simulink model "Simulator"  (R2024a)
settings: Solver=VariableStepAuto  StartTime=0.0  StopTime=inf  RelTol=1e-5
values from neighbouring files (symbols this model uses):
  I = [3000 0 0 ... (first row only)    [Constants_gui.m]    (also in constants.m; mbi.m = [15, .25, .20; set_up_HW7.m = I-Id; setupConstantRateSDA.m)
  invI = inv(I)    [Constants_gui.m]    (also in constants.m; mbi.m; set_up_HW7.m; setupConstantRateSDA.m)
  q_init = q_init/norm(q_init)    [Constants_gui.m]    (also in constants.m = [-0.5 -0.5 -0.5 0.5]; mbi.m = [0 0 0 1]'; set_up_HW7.m = [0 0 0 1]'; setupConstantRateSDA.m)
  wbn_init = pi/30*[0 0 0]'    [Constants_gui.m]    (also in constants.m = pi/180 * [0.1; 0.2; 0.15]; mbi.m = [0 0 0]'; set_up_HW7.m = pi/30*[0 0 .01]'; setupConstantRateSDA.m)
  wn = 0.01    [Constants_gui.m]    (also in constants.m = 0.05; setupConstantRateSDA.m = 0.05)
  zet = .7071    (= 0.7071)    [Constants_gui.m]    (also in constants.m; setupConstantRateSDA.m)
undefined symbols (not defined in the file or in its folder): w_init
libraries: sharedtransform x6, aerolibutil x5, sharedutil x2, simulink x2, dspinverses x1
(part 3 of 4)

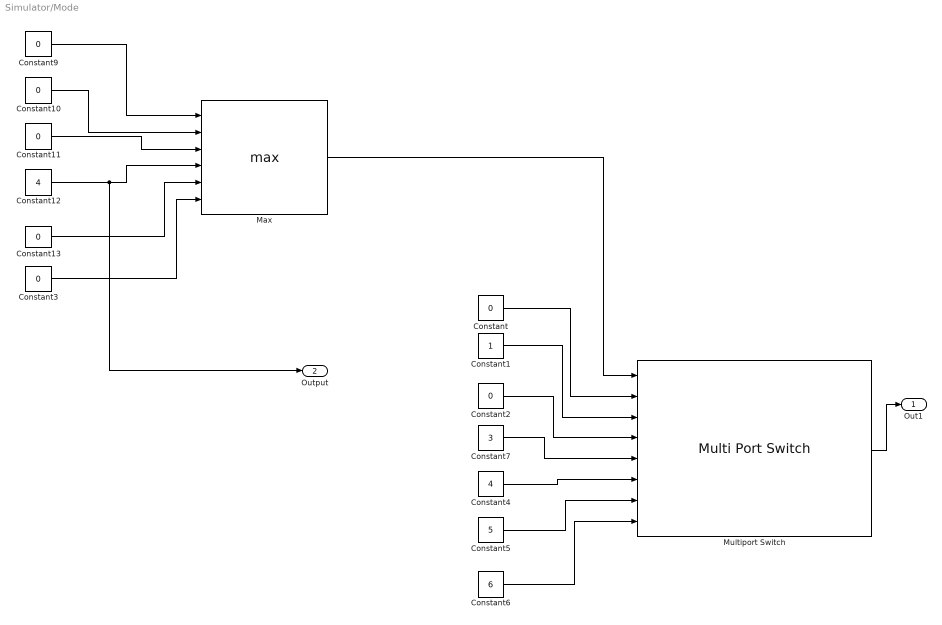
== system Simulator/Mode ==
  Constant{,2..3,9..11,13} (7 alike) : Constant  Value=0
  Constant1 : Constant
  Constant12 : Constant  Value=4
  Constant4 : Constant  Value=4
  Constant5 : Constant  Value=5
  Constant6 : Constant  Value=6
  Constant7 : Constant  Value=3
  Max : MinMax  Function=max  Inputs=6
  Multiport Switch : MultiPortSwitch  DataPortOrder=Specify indices  Inputs=6  DataPortIndices={0,1,2,3,4,5,6}  SaturateOnIntegerOverflow=off  InputSameDT=off
  Out1 : Outport
  Output : Outport  Port=2
  wires:
  Multiport Switch/1 -> Out1/1
  Constant6/1 -> Multiport Switch/8
  Constant5/1 -> Multiport Switch/7
  Constant4/1 -> Multiport Switch/6
  Constant7/1 -> Multiport Switch/5
  Constant2/1 -> Multiport Switch/4
  Constant1/1 -> Multiport Switch/3
  Constant/1 -> Multiport Switch/2
  Constant9/1 -> Max/1
  Constant10/1 -> Max/2
  Constant11/1 -> Max/3
  Constant12/1 -> Output/1, Max/4
  Constant13/1 -> Max/5
  Constant3/1 -> Max/6
  Max/1 -> Multiport Switch/1

== system Simulator/Mode 0  ==
  In1 : Inport
  In2 : Inport  Port=2
  Q : Inport  Port=3
  Rate : Inport  Port=4
  Commanded Quaternion : Subsystem
  Constant : Constant
  Switch : Switch  Criteria=u2 > Threshold  SaturateOnIntegerOverflow=off  InputSameDT=off
  Rate2 : Outport
  Quaternion : Outport  Port=2
  wires:
  Rate/1 -> Rate2/1
  Switch/1 -> Quaternion/1
  Constant/1 -> Switch/2
  Q/1 -> Switch/3
  Commanded Quaternion/1(QUaternion) -> Switch/1

== system Simulator/Mode 1: Full Test ==
  In1 : Inport
  Out1 : Outport
  Out2 : Outport  Port=2
  wires:
  In1/1 -> Out2/1, Out1/1

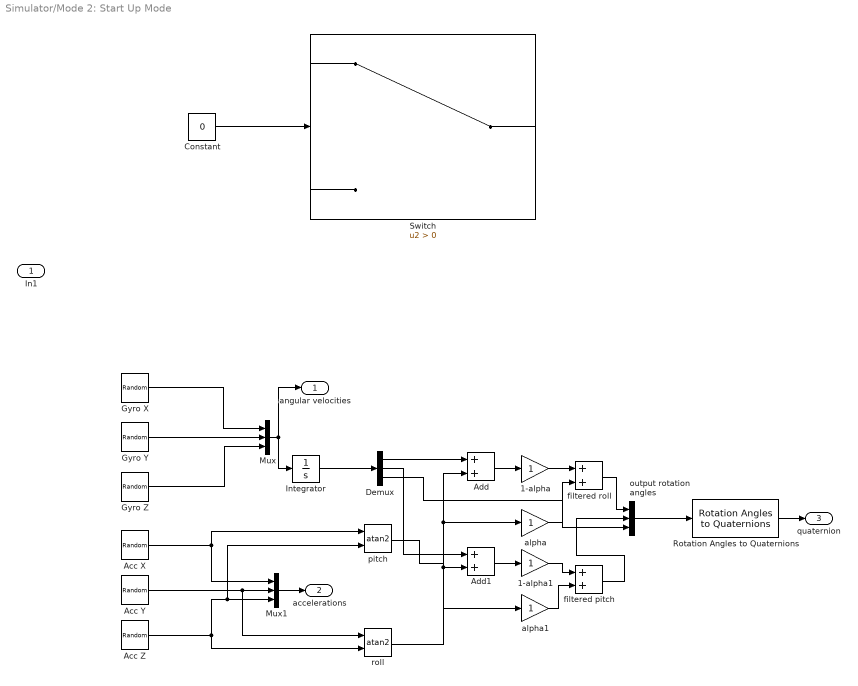
== system Simulator/Mode 2: Start Up Mode ==
  In1 : Inport
  1-alpha : Gain
  1-alpha1 : Gain
  Acc X : UniformRandomNumber  Minimum=w_init  Maximum=100  SampleTime=0.1
  Acc Y : UniformRandomNumber  Minimum=w_init  Maximum=100  SampleTime=0.1
  Acc Z : UniformRandomNumber  Minimum=w_init  Maximum=100  SampleTime=0.1
  Add : Sum
  Add1 : Sum
  Constant : Constant  Value=0
  Demux : Demux  Outputs=3
  Gyro X : UniformRandomNumber  Minimum=w_init  Maximum=100  SampleTime=0.1
  Gyro Y : UniformRandomNumber  Minimum=w_init  Maximum=100  SampleTime=0.1
  Gyro Z : UniformRandomNumber  Minimum=w_init  Maximum=100  SampleTime=0.1
  Integrator : Integrator
  Mux : Mux  Inputs=3
  Mux1 : Mux  Inputs=3
  Rotation Angles to Quaternions : sharedtransform/Rotation Angles to Quaternions  rotationOrder=XYZ  aMode=aMode
  Switch : Switch  Criteria=u2 > Threshold  SaturateOnIntegerOverflow=off  InputSameDT=off
  alpha : Gain
  alpha1 : Gain
  filtered pitch : Sum
  filtered roll : Sum
  output rotation angles : Mux  Inputs=3
  pitch : Trigonometry  Operator=atan2
  roll : Trigonometry  Operator=atan2
  angular velocities : Outport
  accelerations : Outport  Port=2
  quaternion : Outport  Port=3
  wires:
  Gyro X/1 -> Mux/1
  Gyro Y/1 -> Mux/2
  Gyro Z/1 -> Mux/3
  Mux/1 -> Integrator/1, angular velocities/1
  Mux1/1 -> accelerations/1
  Acc X/1 -> pitch/1, Mux1/1
  Acc Y/1 -> Mux1/2, roll/1
  Acc Z/1 -> roll/2, Mux1/3, pitch/2
  Integrator/1 -> Demux/1
  Demux/3 -> output rotation angles/3
  Demux/1 -> Add/1
  roll/1 -> alpha/1, Add/2
  Add/1 -> 1-alpha/1
  1-alpha/1 -> filtered roll/1
  alpha/1 -> filtered roll/2
  Demux/2 -> Add1/1
  pitch/1 -> Add1/2, alpha1/1
  Add1/1 -> 1-alpha1/1
  1-alpha1/1 -> filtered pitch/1
  alpha1/1 -> filtered pitch/2
  filtered roll/1 -> output rotation angles/1
  filtered pitch/1 -> output rotation angles/2
  output rotation angles/1 -> Rotation Angles to Quaternions/1
  Rotation Angles to Quaternions/1 -> quaternion/1
  Constant/1 -> Switch/2

== system Simulator/Mode 3: Constant Rate ==
  rotation rate mode : Inport
  commanded Velocity : Inport  Port=2
  "Free Rigid Body " : Subsystem
  Kd1 : Gain  Gain=2 * zet * wn * I  Multiplication=Matrix(K*u)  SaturateOnIntegerOverflow=on  OutDataTypeStr=Inherit: Same as input  ParamDataTypeStr=Inherit: Same as input
  Sum1 : Sum  Inputs=|+-
  rotation rate : Outport
  "quaat " : Outport  Port=2
  wires:
  Kd1/1 -> "Free Rigid Body "/1(In2)
  Sum1/1 -> Kd1/1
  "Free Rigid Body "/2(w) -> rotation rate/1, Sum1/2
  "Free Rigid Body "/1(q) -> "quaat "/1
  commanded Velocity/1 -> Sum1/1

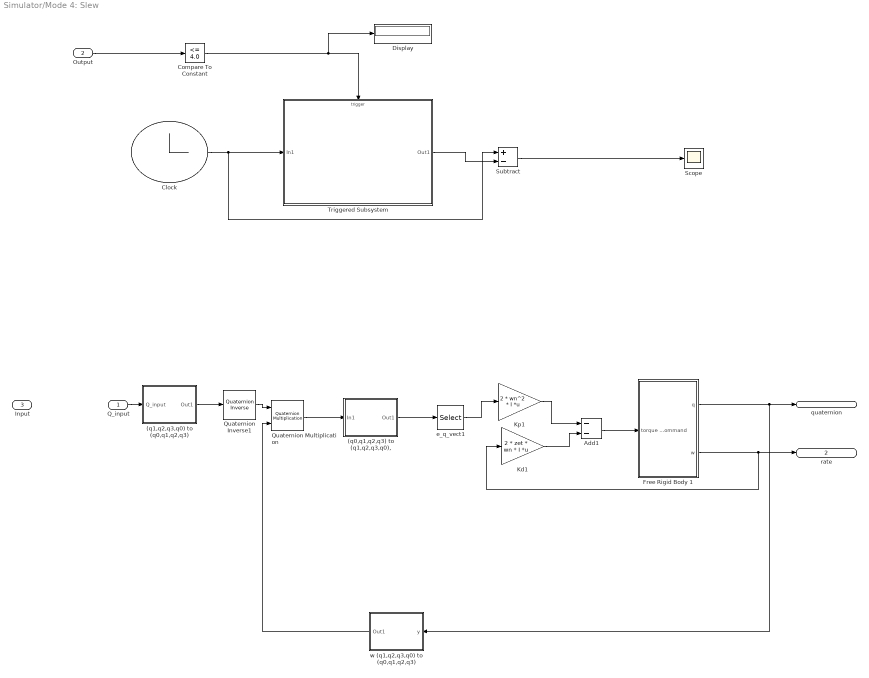
== system Simulator/Mode 4: Slew ==
  Q_input : Inport
  Output : Inport  Port=2
  " Input" : Inport  Port=3
  (q0,q1,q2,q3) to (q1,q2,q3,q0), : Subsystem
  "(q1,q2,q3,q0) to (q0,q1,q2,q3) " : Subsystem
  Add1 : Sum  Inputs=--
  Clock : Clock
  Compare To Constant : simulink/Logic and Bit Operations/Compare To Constant  relop=<=  const=4.0  OutDataTypeStr=boolean
  Display : Display
  Free Rigid Body 1 : Subsystem
  Kd1 : Gain  Gain=2 * zet * wn * I  Multiplication=Matrix(K*u)  SaturateOnIntegerOverflow=on  OutDataTypeStr=Inherit: Same as input  ParamDataTypeStr=Inherit: Same as input
  Kp1 : Gain  Gain=2 * wn^2 * I  Multiplication=Matrix(K*u)  SaturateOnIntegerOverflow=on  OutDataTypeStr=Inherit: Same as input  ParamDataTypeStr=Inherit: Same as input
  Quaternion Inverse1 : aerolibutil/Quaternion Inverse
  Quaternion Multiplication : aerolibutil/Quaternion Multiplication
  Scope : Scope
  Subtract : Sum  Inputs=+-
  Triggered Subsystem : Subsystem  TreatAsAtomicUnit=on
  e_q_vect1 : Selector  InputPortWidth=4  IndexOptions=Index vector (dialog)  Indices=[1 2 3]  OutputSizes=1
  "w (q1,q2,q3,q0) to (q0,q1,q2,q3) " : Subsystem
      settings: PortSchema="{\"entries\":[{\"content\":{\"sides\":[{\"content\":{\"connectorIds\":[\"Out1\"]},\"type\":\"ConnectorPlacement.EquallySpacedRectSide\",\"uuid\":\"97b477ad-5663-4010-b344-d27b8ec095be\"},{\"content\":{\"connectorIds\":[\"In1\"],\"side\":\"RIGHT\"},\"type\":\"ConnectorPlacement.EquallySpacedRectSide\",\"uuid\":\"41fe4029-0263-4427-bdfc-3c26258b8a65\"},{\"content\":{\"side\":\"TOP\"},\"type\":\"ConnectorPlacement.EquallySpacedRectSide\",\"uuid\":\"9fb3a03d-539a-4245-bd7d-8174d3d0797f\"}]},\"type\":\"ConnectorPlacement.EquallySpacedConnector\",\"uuid\":\"44222554-f3ae-4bc6-b92c-7571a5ce84f7\"}],\"packageUris\":[\"http://schema.mathworks.com/mf0/Connector/R2020b\"],\"version\":\"1.0\"}"
  quaternion : Outport
  rate : Outport  Port=2
  wires:
  Free Rigid Body 1/2(w) -> rate/1, Kd1/1
  Quaternion Inverse1/1 -> Quaternion Multiplication/1
  (q0,q1,q2,q3) to (q1,q2,q3,q0),/1(Out1) -> e_q_vect1/1
  Quaternion Multiplication/1 -> (q0,q1,q2,q3) to (q1,q2,q3,q0),/1(In1)
  Add1/1 -> Free Rigid Body 1/1(torque command)
  "w (q1,q2,q3,q0) to (q0,q1,q2,q3) "/1(Out1) -> Quaternion Multiplication/2
  "(q1,q2,q3,q0) to (q0,q1,q2,q3) "/1(Out1) -> Quaternion Inverse1/1
  Kd1/1 -> Add1/2
  Free Rigid Body 1/1(q) -> quaternion/1, "w (q1,q2,q3,q0) to (q0,q1,q2,q3) "/1(y)
  e_q_vect1/1 -> Kp1/1
  Kp1/1 -> Add1/1
  Q_input/1 -> "(q1,q2,q3,q0) to (q0,q1,q2,q3) "/1(Q_input)
  Clock/1 -> Subtract/1, Triggered Subsystem/1(In1)
  Output/1 -> Compare To Constant/1
  Compare To Constant/1 -> Display/1, Triggered Subsystem/Trigger
  Triggered Subsystem/1(Out1) -> Subtract/2
  Subtract/1 -> Scope/1

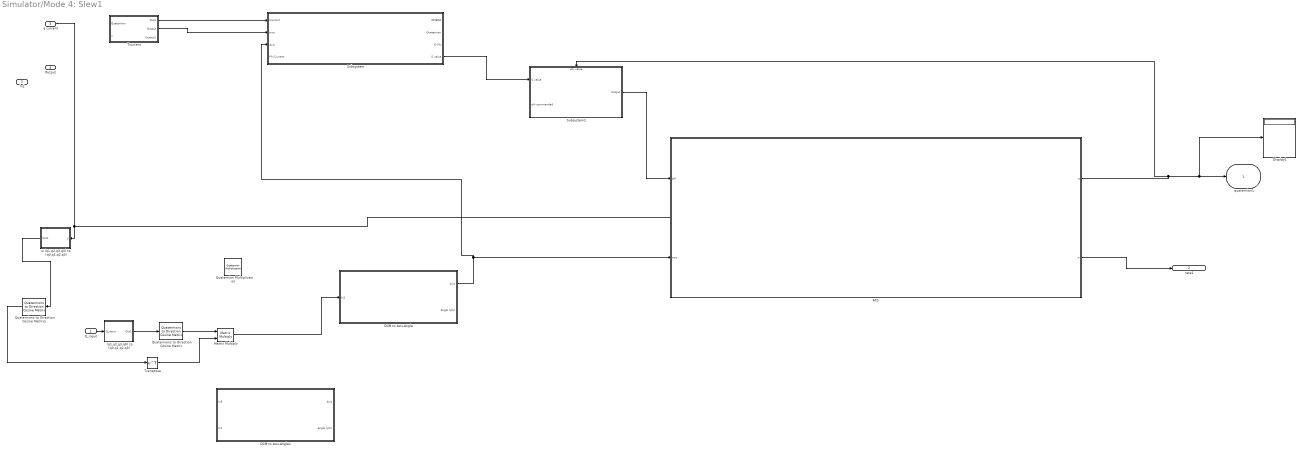
== system Simulator/Mode 4: Slew1 ==
  Q_input : Inport
  In2 : Inport  Port=2
  q current : Inport  Port=3
  Output : Inport  Port=4
  "(q1,q2,q3,q0) to (q0,q1,q2,q3) " : Subsystem
  ACS : Subsystem
  DCM to Axis-Angle : Subsystem
  DCM to Axis-Angle1 : Subsystem
  Display1 : Display
  Matrix Multiply : Product  Multiplication=Matrix(*)
  Quaternion Multiplication : aerolibutil/Quaternion Multiplication
  Quaternions to Direction Cosine Matrix : sharedtransform/Quaternions to  Direction Cosine Matrix  aMode=aMode
      settings: LibrarySourceBlock=|
      | aerolibtransform2/Quaternions to
      | Direction Cosine Matrix
  Quaternions to Direction Cosine Matrix1 : sharedtransform/Quaternions to  Direction Cosine Matrix  aMode=aMode
      settings: LibrarySourceBlock=|
      | aerolibtransform2/Quaternions to
      | Direction Cosine Matrix
  Subsystem : Subsystem
  Subsystem2 : Subsystem
      settings: PortSchema="{\"entries\":[{\"content\":{\"sides\":[{\"content\":{\"connectorIds\":[\"In1\",\"In2\"]},\"type\":\"ConnectorPlacement.EquallySpacedRectSide\",\"uuid\":\"d1e910e7-02fe-476a-80f5-06936a5c67bc\"},{\"content\":{\"connectorIds\":[\"Out1\"],\"side\":\"RIGHT\"},\"type\":\"ConnectorPlacement.EquallySpacedRectSide\",\"uuid\":\"f2ee99f2-c038-4b18-8075-388ccc728d71\"},{\"content\":{\"connectorIds\":[\"In3\"],\"side\":\"TOP\"},\"type\":\"ConnectorPlacement.EquallySpacedRectSide\",\"uuid\":\"7923cf94-d68b-4fff-9236-03f2ad3fb038\"}]},\"type\":\"ConnectorPlacement.EquallySpacedConnector\",\"uuid\":\"859f0eee-a4bc-4454-90a5-75b168cd4378\"}],\"packageUris\":[\"http://schema.mathworks.com/mf0/Connector/R2020b\"],\"version\":\"1.0\"}"
  Tcurrent : Subsystem
  Transpose : Math  Operator=transpose
  "w (q1,q2,q3,q0) to (q0,q1,q2,q3) " : Subsystem
      settings: PortSchema="{\"entries\":[{\"content\":{\"sides\":[{\"content\":{\"connectorIds\":[\"Out1\"]},\"type\":\"ConnectorPlacement.EquallySpacedRectSide\",\"uuid\":\"97b477ad-5663-4010-b344-d27b8ec095be\"},{\"content\":{\"connectorIds\":[\"In1\"],\"side\":\"RIGHT\"},\"type\":\"ConnectorPlacement.EquallySpacedRectSide\",\"uuid\":\"41fe4029-0263-4427-bdfc-3c26258b8a65\"},{\"content\":{\"side\":\"TOP\"},\"type\":\"ConnectorPlacement.EquallySpacedRectSide\",\"uuid\":\"9fb3a03d-539a-4245-bd7d-8174d3d0797f\"}]},\"type\":\"ConnectorPlacement.EquallySpacedConnector\",\"uuid\":\"44222554-f3ae-4bc6-b92c-7571a5ce84f7\"}],\"packageUris\":[\"http://schema.mathworks.com/mf0/Connector/R2020b\"],\"version\":\"1.0\"}"
  quaternion1 : Outport
  rate1 : Outport  Port=2
  wires:
  Q_input/1 -> "(q1,q2,q3,q0) to (q0,q1,q2,q3) "/1(Q_input)
  Transpose/1 -> Matrix Multiply/2
  "w (q1,q2,q3,q0) to (q0,q1,q2,q3) "/1(Out1) -> Quaternions to Direction Cosine Matrix1/1
  Tcurrent/1(Out1) -> Subsystem/1(tcurrent)
  Tcurrent/2(Output) -> Subsystem/2(tnot)
  Quaternions to Direction Cosine Matrix/1 -> Matrix Multiply/1
  Matrix Multiply/1 -> DCM to Axis-Angle/1(In1)
  DCM to Axis-Angle/1(Axis) -> Subsystem/3(Axis), ACS/2(axis)
  Quaternions to Direction Cosine Matrix1/1 -> Transpose/1
  ACS/1(q) -> Subsystem2/3(phi value), Display1/1, quaternion1/1
  ACS/2(w) -> rate1/1
  q current/1 -> "w (q1,q2,q3,q0) to (q0,q1,q2,q3) "/1(y)
  Subsystem/4(S value) -> Subsystem2/1(S value)
  "(q1,q2,q3,q0) to (q0,q1,q2,q3) "/1(Out1) -> Quaternions to Direction Cosine Matrix/1
  Subsystem2/1(Output) -> ACS/1(phi)
  ? -> DCM to Axis-Angle1/1(In3)
  ? -> DCM to Axis-Angle1/2(In1)

== system Simulator/Mode 5: Attitude Control ==
  In2 : Inport
  Q_input : Inport  Port=2
  Add : Sum  Inputs=+-
  "Free Rigid Body " : Subsystem
  Kd : Gain  Gain=2 * zet * wn * I  Multiplication=Matrix(K*u)  SaturateOnIntegerOverflow=on  OutDataTypeStr=Inherit: Same as input  ParamDataTypeStr=Inherit: Same as input
  Kp : Gain  Gain=2 * wn^2 * I  Multiplication=Matrix(K*u)  SaturateOnIntegerOverflow=on  OutDataTypeStr=Inherit: Same as input  ParamDataTypeStr=Inherit: Same as input
  Sum : Sum  Inputs=|+-
  e_q_vect : Selector  InputPortWidth=4  IndexOptions=Index vector (dialog)  Indices=[1 2 3]  OutputSizes=1
  quaternion : Outport
  rate : Outport  Port=2
  wires:
  Kp/1 -> Add/1
  Sum/1 -> e_q_vect/1
  "Free Rigid Body "/1(q) -> quaternion/1, Sum/2
  e_q_vect/1 -> Kp/1
  Kd/1 -> Add/2
  "Free Rigid Body "/2(w) -> rate/1, Kd/1
  Add/1 -> "Free Rigid Body "/1(torque command)
  Q_input/1 -> Sum/1

== system Simulator/Mode 6: Momentum Dump ==
  In1 : Inport
  In2 : Inport  Port=2
  Cross : Subsystem
  F_thrusters : Constant
  Gain : Gain  Gain=-1
  I_sc : Constant  Value=I
  Matrix Divide : Product  Inputs=*/  Multiplication=Matrix(*)
  current angular momentum : Product  Multiplication=Matrix(*)
  r_thrusters : Constant
  commanded thrust time : Outport
  wires:
  I_sc/1 -> current angular momentum/1
  Gain/1 -> Matrix Divide/1
  Cross/1(AxB) -> Matrix Divide/2
  Matrix Divide/1 -> commanded thrust time/1
  current angular momentum/1 -> Gain/1
  In2/1 -> current angular momentum/2
  r_thrusters/1 -> Cross/1(A)
  F_thrusters/1 -> Cross/2(B)

== system Simulator/Subsystem ==
  q : Inport
  " 1" : Demux  Outputs=3
      settings: DisplayOption=none
  " 2" : Demux  Outputs=3
      settings: DisplayOption=none
  Display{,1..3} (4 alike) : Display
  Mux : Mux  Inputs=2
  Quaternions to Rotation Angles : sharedtransform/Quaternions to Rotation Angles  rotationOrder=ZYX  aMode=aMode
  Quaternions to Rotation Angles1 : sharedtransform/Quaternions to Rotation Angles  rotationOrder=ZYX  aMode=aMode
  wires:
  " 2"/3 -> Display2/1
  Quaternions to Rotation Angles/1 -> " 2"/1
  " 2"/2 -> Display1/1
  q/1 -> Quaternions to Rotation Angles1/1, Quaternions to Rotation Angles/1
  " 2"/1 -> Display/1
  Quaternions to Rotation Angles1/1 -> " 1"/1
  " 1"/1 -> Mux/1
  " 1"/3 -> Mux/2
  Mux/1 -> Display3/1

== system Simulator/Commanded values/Commanded Quaternion ==
  Constant{,1..3} (4 alike) : Constant  Value=0.5
  Vector Concatenate : Concatenate  NumInputs=4
  Out1 : Outport
  wires:
  Constant2/1 -> Vector Concatenate/1
  Constant3/1 -> Vector Concatenate/4
  Vector Concatenate/1 -> Out1/1
  Constant1/1 -> Vector Concatenate/3
  Constant/1 -> Vector Concatenate/2

== system Simulator/Commanded values/Commanded Velocity ==
  Constant : Constant  Value=0
  Constant1 : Constant  Value=5
  Constant2 : Constant  Value=0
  Vector Concatenate : Concatenate  NumInputs=3
  Out1 : Outport
  wires:
  Constant/1 -> Vector Concatenate/2
  Constant1/1 -> Vector Concatenate/3
  Vector Concatenate/1 -> Out1/1
  Constant2/1 -> Vector Concatenate/1

== system Simulator/Mode 0 /Commanded Quaternion ==
  Constant : Constant  Value=2
  Constant1 : Constant  Value=3
  Constant2 : Constant
  Constant3 : Constant  Value=4
  Vector Concatenate : Concatenate  NumInputs=4
  QUaternion : Outport
  wires:
  Constant2/1 -> Vector Concatenate/1
  Constant3/1 -> Vector Concatenate/4
  Vector Concatenate/1 -> QUaternion/1
  Constant1/1 -> Vector Concatenate/3
  Constant/1 -> Vector Concatenate/2

== system Simulator/Mode 3: Constant Rate/Free Rigid Body  ==
  In2 : Inport
  Cross : Subsystem
  DCM : ToWorkspace  VariableName=DCM  SaveFormat=Structure With Time  SampleTime=-1
  Inertia : Gain  Gain=I  Multiplication=Matrix(K*u)  SaturateOnIntegerOverflow=on  OutDataTypeStr=Inherit: Same as input  ParamDataTypeStr=Inherit: Same as input
  Isc inverse : Gain  Gain=invI  Multiplication=Matrix(K*u)  SaturateOnIntegerOverflow=on  OutDataTypeStr=Inherit: Same as input  ParamDataTypeStr=Inherit: Same as input
  Quaternion Integration : Subsystem
  Subsystem : Subsystem
  Sum : Sum  Inputs=|+-  InputSameDT=on  SaturateOnIntegerOverflow=on  OutDataTypeStr=Inherit: Same as first input
  quat : ToWorkspace  VariableName=quat  SaveFormat=Structure With Time  SampleTime=-1
  "wdot -> w" : Integrator  InitialCondition=wbn_init
  q : Outport
  w : Outport  Port=2
  wires:
  Isc inverse/1 -> "wdot -> w"/1
  "wdot -> w"/1 -> w/1, Quaternion Integration/1(w_Body), Inertia/1, Cross/1(A)
  Sum/1 -> Isc inverse/1
  Cross/1(AxB) -> Sum/2
  Inertia/1 -> Cross/2(B)
  Quaternion Integration/1(q_I_Body) -> Subsystem/1(q1 q2 q3 q4), q/1, quat/1
  Subsystem/1(DCM) -> DCM/1
  In2/1 -> Sum/1

== system Simulator/Mode 4: Slew/(q0,q1,q2,q3) to (q1,q2,q3,q0), ==
  In1 : Inport
  Display : Display
  Display1 : Display
  Vector Concatenate : Concatenate
  e_q_vect1 : Selector  InputPortWidth=4  IndexOptions=Index vector (dialog)  Indices=[2 3 4]  OutputSizes=1
  e_q_vect2 : Selector  InputPortWidth=4  IndexOptions=Index vector (dialog)  Indices=[1]  OutputSizes=1
  Out1 : Outport
  wires:
  Vector Concatenate/1 -> Display1/1, Out1/1
  In1/1 -> Display/1, e_q_vect2/1, e_q_vect1/1
  e_q_vect1/1 -> Vector Concatenate/1
  e_q_vect2/1 -> Vector Concatenate/2

== system Simulator/Mode 4: Slew/(q1,q2,q3,q0) to (q0,q1,q2,q3)  ==
  Q_input : Inport
  Quaternion Normalize : sharedutil/Quaternion Normalize  aMode=aMode
  Vector Concatenate : Concatenate
  e_q_vect1 : Selector  InputPortWidth=4  IndexOptions=Index vector (dialog)  Indices=[1 2 3]  OutputSizes=1
  e_q_vect2 : Selector  InputPortWidth=4  IndexOptions=Index vector (dialog)  Indices=[4]  OutputSizes=1
  Out1 : Outport
  wires:
  Q_input/1 -> e_q_vect2/1, e_q_vect1/1
  e_q_vect2/1 -> Vector Concatenate/1
  e_q_vect1/1 -> Vector Concatenate/2
  Vector Concatenate/1 -> Quaternion Normalize/1
  Quaternion Normalize/1 -> Out1/1

== system Simulator/Mode 4: Slew/Free Rigid Body 1 ==
  torque command : Inport
  Cross : Subsystem
  DCM : ToWorkspace  Commented=on  VariableName=DCM  SaveFormat=Structure With Time  SampleTime=-1
  Inertia : Gain  Gain=I  Multiplication=Matrix(K*u)  SaturateOnIntegerOverflow=on  OutDataTypeStr=Inherit: Same as input  ParamDataTypeStr=Inherit: Same as input
  Isc inverse : Gain  Gain=invI  Multiplication=Matrix(K*u)  SaturateOnIntegerOverflow=on  OutDataTypeStr=Inherit: Same as input  ParamDataTypeStr=Inherit: Same as input
  Quaternion Integration : Subsystem
  Subsystem : Subsystem  Commented=on
  Sum : Sum  Inputs=|+-  InputSameDT=on  SaturateOnIntegerOverflow=on  OutDataTypeStr=Inherit: Same as first input
  "wdot -> w" : Integrator  InitialCondition=wbn_init
  q : Outport
  w : Outport  Port=2
  wires:
  Isc inverse/1 -> "wdot -> w"/1
  "wdot -> w"/1 -> w/1, Quaternion Integration/1(w_Body), Inertia/1, Cross/1(A)
  Sum/1 -> Isc inverse/1
  torque command/1 -> Sum/1
  Cross/1(AxB) -> Sum/2
  Inertia/1 -> Cross/2(B)
  Quaternion Integration/1(q_I_Body) -> Subsystem/1(q1 q2 q3 q4), q/1
  Subsystem/1(DCM) -> DCM/1

== system Simulator/Mode 4: Slew/Triggered Subsystem ==
  In1 : Inport
  Trigger : TriggerPort  VariantControl=(inherit)
  Out1 : Outport
  wires:
  In1/1 -> Out1/1

== system Simulator/Mode 4: Slew/w (q1,q2,q3,q0) to (q0,q1,q2,q3)  ==
  y : Inport
  Vector Concatenate : Concatenate
  e_q_vect1 : Selector  InputPortWidth=4  IndexOptions=Index vector (dialog)  Indices=[1 2 3]  OutputSizes=1
  e_q_vect2 : Selector  InputPortWidth=4  IndexOptions=Index vector (dialog)  Indices=[4]  OutputSizes=1
  Out1 : Outport
  wires:
  Vector Concatenate/1 -> Out1/1
  e_q_vect1/1 -> Vector Concatenate/2
  e_q_vect2/1 -> Vector Concatenate/1
  y/1 -> e_q_vect1/1, e_q_vect2/1

== system Simulator/Mode 4: Slew1/(q1,q2,q3,q0) to (q0,q1,q2,q3)  ==
  Q_input : Inport
  Quaternion Normalize : sharedutil/Quaternion Normalize  aMode=aMode
  Vector Concatenate : Concatenate
  e_q_vect1 : Selector  InputPortWidth=4  IndexOptions=Index vector (dialog)  Indices=[1 2 3]  OutputSizes=1
  e_q_vect2 : Selector  InputPortWidth=4  IndexOptions=Index vector (dialog)  Indices=[4]  OutputSizes=1
  Out1 : Outport
  wires:
  Quaternion Normalize/1 -> Out1/1
  Vector Concatenate/1 -> Quaternion Normalize/1
  e_q_vect1/1 -> Vector Concatenate/2
  e_q_vect2/1 -> Vector Concatenate/1
  Q_input/1 -> e_q_vect1/1, e_q_vect2/1

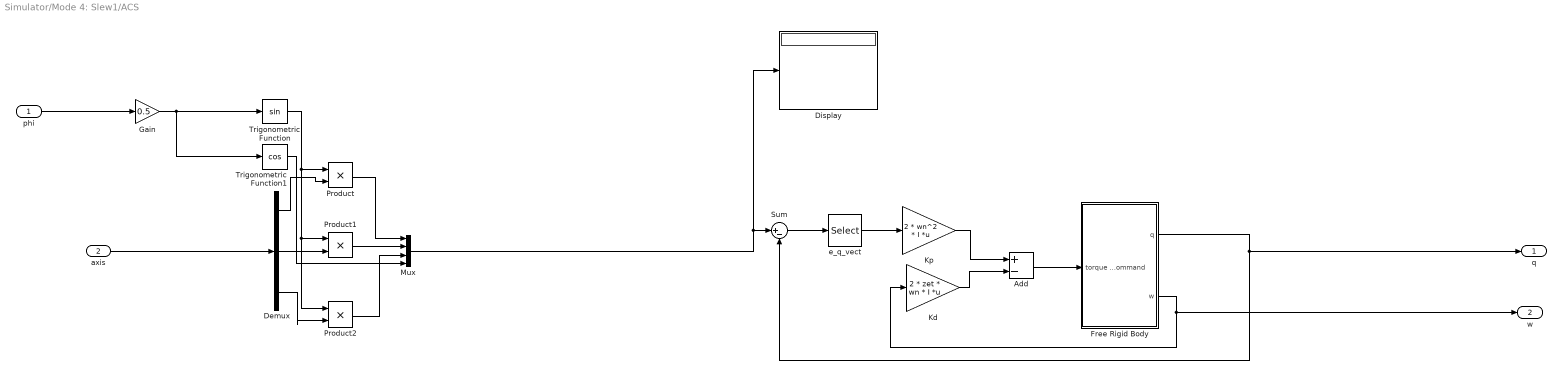
== system Simulator/Mode 4: Slew1/ACS ==
  phi : Inport
  axis : Inport  Port=2
  Add : Sum  Inputs=+-
  Demux : Demux  Outputs=3
  Display : Display
  "Free Rigid Body " : Subsystem
  Gain : Gain  Gain=0.5
  Kd : Gain  Gain=2 * zet * wn * I  Multiplication=Matrix(K*u)  SaturateOnIntegerOverflow=on  OutDataTypeStr=Inherit: Same as input  ParamDataTypeStr=Inherit: Same as input
  Kp : Gain  Gain=2 * wn^2 * I  Multiplication=Matrix(K*u)  SaturateOnIntegerOverflow=on  OutDataTypeStr=Inherit: Same as input  ParamDataTypeStr=Inherit: Same as input
  Mux : Mux
  Product : Product
  Product1 : Product
  Product2 : Product
  Sum : Sum  Inputs=|+-
  Trigonometric Function : Trigonometry
  Trigonometric Function1 : Trigonometry  Operator=cos
  e_q_vect : Selector  InputPortWidth=4  IndexOptions=Index vector (dialog)  Indices=[1 2 3]  OutputSizes=1
  q : Outport
  w : Outport  Port=2
  wires:
  Product1/1 -> Mux/2
  Product2/1 -> Mux/3
  Demux/1 -> Product/2
  Gain/1 -> Trigonometric Function1/1, Trigonometric Function/1
  Product/1 -> Mux/1
  axis/1 -> Demux/1
  phi/1 -> Gain/1
  Demux/2 -> Product1/2
  Demux/3 -> Product2/2
  Trigonometric Function1/1 -> Mux/4
  Trigonometric Function/1 -> Product2/1, Product1/1, Product/1
  Kp/1 -> Add/1
  "Free Rigid Body "/2(w) -> w/1, Kd/1
  e_q_vect/1 -> Kp/1
  "Free Rigid Body "/1(q) -> q/1, Sum/2
  Kd/1 -> Add/2
  Sum/1 -> e_q_vect/1
  Add/1 -> "Free Rigid Body "/1(torque command)
  Mux/1 -> Display/1, Sum/1

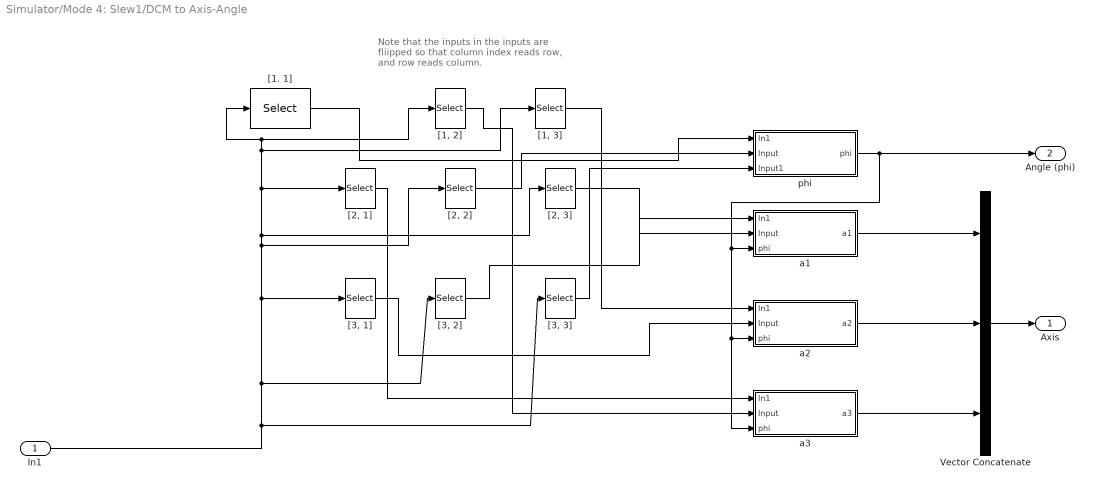
== system Simulator/Mode 4: Slew1/DCM to Axis-Angle ==
  note: Note that the inputs in the inputs are fliipped so that column index reads row, and row reads column.
  In1 : Inport
  Vector Concatenate : Concatenate  NumInputs=3
  "[1, 2]" : Selector  NumberOfDimensions=2  InputPortWidth=3  IndexOptions=Index vector (dialog),Index vector (dialog)  Indices=2,1  OutputSizes=1,1
  "[1, 3]" : Selector  NumberOfDimensions=2  InputPortWidth=3  IndexOptions=Index vector (dialog),Index vector (dialog)  Indices=3,1  OutputSizes=1,1
  "[1. 1]" : Selector  NumberOfDimensions=2  InputPortWidth=3  IndexOptions=Index vector (dialog),Index vector (dialog)  Indices=1,1  OutputSizes=1,1
  "[2, 1]" : Selector  NumberOfDimensions=2  InputPortWidth=3  IndexOptions=Index vector (dialog),Index vector (dialog)  Indices=1,2  OutputSizes=1,1
  "[2, 2]" : Selector  NumberOfDimensions=2  InputPortWidth=3  IndexOptions=Index vector (dialog),Index vector (dialog)  Indices=2,2  OutputSizes=1,1
  "[2, 3]" : Selector  NumberOfDimensions=2  InputPortWidth=3  IndexOptions=Index vector (dialog),Index vector (dialog)  Indices=3,2  OutputSizes=1,1
  "[3, 1]" : Selector  NumberOfDimensions=2  InputPortWidth=3  IndexOptions=Index vector (dialog),Index vector (dialog)  Indices=1,3  OutputSizes=1,1
  "[3, 2]" : Selector  NumberOfDimensions=2  InputPortWidth=3  IndexOptions=Index vector (dialog),Index vector (dialog)  Indices=2,3  OutputSizes=1,1
  "[3, 3]" : Selector  NumberOfDimensions=2  InputPortWidth=3  IndexOptions=Index vector (dialog),Index vector (dialog)  Indices=3,3  OutputSizes=1,1
  a1 : Subsystem
  a2 : Subsystem
  a3 : Subsystem
  phi : Subsystem
  Axis : Outport
  Angle (phi) : Outport  Port=2
  wires:
  Vector Concatenate/1 -> Axis/1
  "[3, 3]"/1 -> phi/3(Input1)
  "[2, 3]"/1 -> a1/2(Input)
  "[1, 3]"/1 -> a2/1(In1)
  a2/1(a2) -> Vector Concatenate/2
  phi/1(phi) -> Angle (phi)/1, a3/3(phi), a2/3(phi), a1/3(phi)
  "[2, 2]"/1 -> phi/2(Input)
  "[1, 2]"/1 -> a3/2(Input)
  "[1. 1]"/1 -> phi/1(In1)
  "[2, 1]"/1 -> a3/1(In1)
  "[3, 1]"/1 -> a2/2(Input)
  "[3, 2]"/1 -> a1/1(In1)
  In1/1 -> "[3, 2]"/1, "[3, 1]"/1, "[2, 1]"/1, "[1, 3]"/1, "[1, 2]"/1, "[1. 1]"/1, "[2, 3]"/1, "[2, 2]"/1, "[3, 3]"/1
  a3/1(a3) -> Vector Concatenate/3
  a1/1(a1) -> Vector Concatenate/1

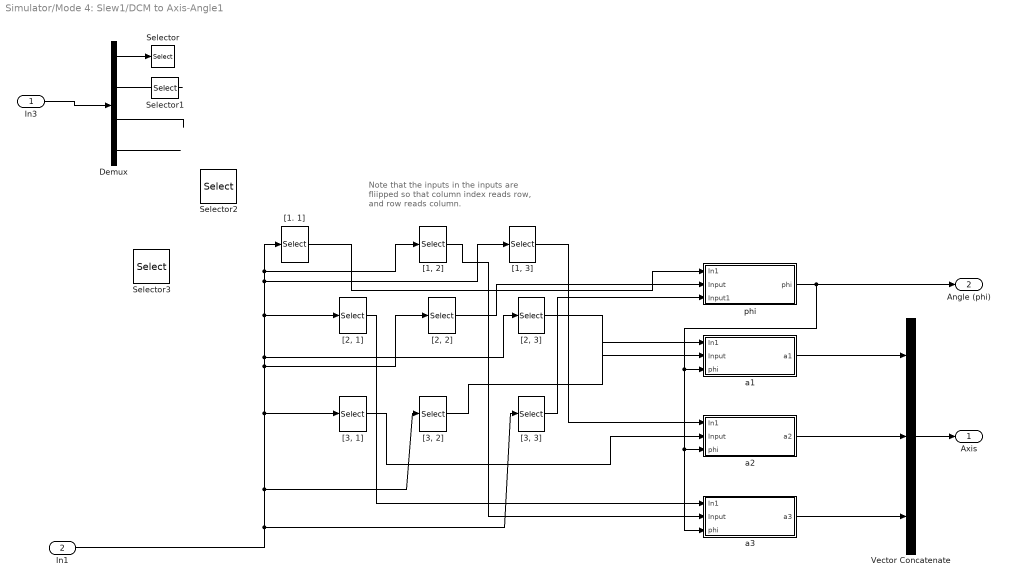
== system Simulator/Mode 4: Slew1/DCM to Axis-Angle1 ==
  note: Note that the inputs in the inputs are fliipped so that column index reads row, and row reads column.
  In3 : Inport
  In1 : Inport  Port=2
  Demux : Demux
  Selector : Selector  InputPortWidth=3  IndexOptions=Index vector (dialog)  Indices=[1 1]  OutputSizes=1
  Selector1 : Selector  InputPortWidth=3  IndexOptions=Index vector (dialog)  Indices=[1 2]  OutputSizes=1
  Selector2 : Selector  InputPortWidth=3  IndexOptions=Index vector (dialog)  Indices=[1 1]  OutputSizes=1
  Selector3 : Selector  InputPortWidth=3  IndexOptions=Index vector (dialog)  Indices=[1 1]  OutputSizes=1
  Vector Concatenate : Concatenate  NumInputs=3
  "[1, 2]" : Selector  NumberOfDimensions=2  InputPortWidth=3  IndexOptions=Index vector (dialog),Index vector (dialog)  Indices=2,1  OutputSizes=1,1
  "[1, 3]" : Selector  NumberOfDimensions=2  InputPortWidth=3  IndexOptions=Index vector (dialog),Index vector (dialog)  Indices=3,1  OutputSizes=1,1
  "[1. 1]" : Selector  NumberOfDimensions=2  InputPortWidth=3  IndexOptions=Index vector (dialog),Index vector (dialog)  Indices=1,1  OutputSizes=1,1
  "[2, 1]" : Selector  NumberOfDimensions=2  InputPortWidth=3  IndexOptions=Index vector (dialog),Index vector (dialog)  Indices=1,2  OutputSizes=1,1
  "[2, 2]" : Selector  NumberOfDimensions=2  InputPortWidth=3  IndexOptions=Index vector (dialog),Index vector (dialog)  Indices=2,2  OutputSizes=1,1
  "[2, 3]" : Selector  NumberOfDimensions=2  InputPortWidth=3  IndexOptions=Index vector (dialog),Index vector (dialog)  Indices=3,2  OutputSizes=1,1
  "[3, 1]" : Selector  NumberOfDimensions=2  InputPortWidth=3  IndexOptions=Index vector (dialog),Index vector (dialog)  Indices=1,3  OutputSizes=1,1
  "[3, 2]" : Selector  NumberOfDimensions=2  InputPortWidth=3  IndexOptions=Index vector (dialog),Index vector (dialog)  Indices=2,3  OutputSizes=1,1
  "[3, 3]" : Selector  NumberOfDimensions=2  InputPortWidth=3  IndexOptions=Index vector (dialog),Index vector (dialog)  Indices=3,3  OutputSizes=1,1
  a1 : Subsystem
  a2 : Subsystem
  a3 : Subsystem
  phi : Subsystem
  Axis : Outport
  Angle (phi) : Outport  Port=2
  wires:
  a1/1(a1) -> Vector Concatenate/1
  a3/1(a3) -> Vector Concatenate/3
  In1/1 -> "[3, 3]"/1, "[2, 2]"/1, "[2, 3]"/1, "[1. 1]"/1, "[1, 2]"/1, "[1, 3]"/1, "[2, 1]"/1, "[3, 1]"/1, "[3, 2]"/1
  "[3, 2]"/1 -> a1/1(In1)
  "[3, 1]"/1 -> a2/2(Input)
  "[2, 1]"/1 -> a3/1(In1)
  "[1. 1]"/1 -> phi/1(In1)
  "[1, 2]"/1 -> a3/2(Input)
  "[2, 2]"/1 -> phi/2(Input)
  phi/1(phi) -> a1/3(phi), a2/3(phi), a3/3(phi), Angle (phi)/1
  a2/1(a2) -> Vector Concatenate/2
  "[1, 3]"/1 -> a2/1(In1)
  "[2, 3]"/1 -> a1/2(Input)
  "[3, 3]"/1 -> phi/3(Input1)
  Vector Concatenate/1 -> Axis/1
  In3/1 -> Demux/1
  Demux/2 -> ?
  Demux/3 -> ?
  Demux/4 -> ?
  Demux/1 -> Selector/1

== system Simulator/Mode 4: Slew1/Subsystem ==
  tcurrent : Inport
  tnot : Inport  Port=2
  Axis : Inport  Port=3
  Phi Current : Inport  Port=4
  Divide : Product  Inputs=*/
  Integrator : Integrator  Commented=on
  Quaternion Integration : Subsystem  Commented=on
  S : Subsystem
  T : Constant  Value=10
  acceleration : Subsystem  Commented=on
  invI : Gain  Commented=on  Gain=invI  Multiplication=Matrix(K*u)
  OMEGA : Outport
  Quaternion : Outport  Port=2
  D Phi : Outport  Port=3
  S value : Outport  Port=4
  wires:
  S/1(Out1) -> S value/1
  Integrator/1 -> Quaternion Integration/1(w_Body), OMEGA/1
  Quaternion Integration/1(q_I_Body) -> Quaternion/1
  Phi Current/1 -> acceleration/4(phi current), Divide/1
  tcurrent/1 -> acceleration/3(tcurrent)
  tnot/1 -> S/1(Input), acceleration/2(tnot)
  Axis/1 -> acceleration/5(Axis)
  invI/1 -> Integrator/1
  acceleration/1(Spacecraft torque) -> invI/1
  T/1 -> Divide/2
  Divide/1 -> D Phi/1

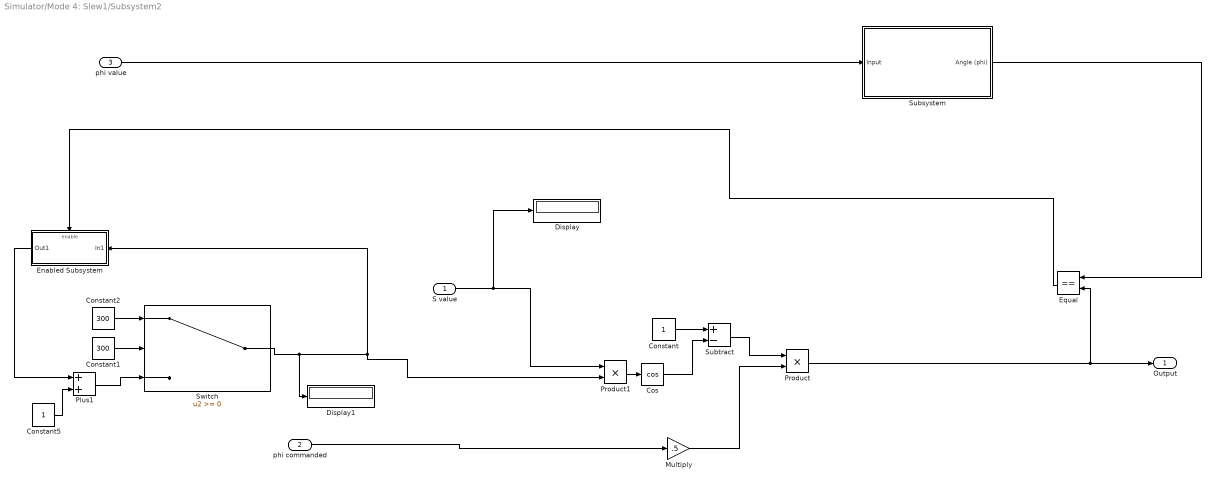
== system Simulator/Mode 4: Slew1/Subsystem2 ==
  S value : Inport
  phi commanded : Inport  Port=2
  phi value : Inport  Port=3
  Constant : Constant
  Constant1 : Constant  Value=300
  Constant2 : Constant  Value=300
  Constant5 : Constant
  Cos : Trigonometry  Operator=cos
  Display : Display
  Display1 : Display
  Enabled Subsystem : Subsystem  TreatAsAtomicUnit=on
  Equal : RelationalOperator  Operator===  OutDataTypeStr=boolean  RndMeth=Simplest  InputSameDT=off
  Multiply : Gain  Gain=.5
  Plus1 : Sum
  Product : Product
  Product1 : Product
  Subsystem : Subsystem
  Subtract : Sum  Inputs=+-
  Switch : Switch  ZeroCross=off  SaturateOnIntegerOverflow=off  InputSameDT=off
  Output : Outport
  wires:
  Equal/1 -> Enabled Subsystem/Enable
  Constant2/1 -> Switch/1
  Constant1/1 -> Switch/2
  Subsystem/1(Angle (phi)) -> Equal/1
  Plus1/1 -> Switch/3
  Enabled Subsystem/1(Out1) -> Plus1/1
  Constant5/1 -> Plus1/2
  phi value/1 -> Subsystem/1(Input)
  Product1/1 -> Cos/1
  Constant/1 -> Subtract/1
  Cos/1 -> Subtract/2
  Subtract/1 -> Product/1
  phi commanded/1 -> Multiply/1
  Multiply/1 -> Product/2
  Product/1 -> Equal/2, Output/1
  S value/1 -> Display/1, Product1/1
  Switch/1 -> Display1/1, Enabled Subsystem/1(In1), Product1/2

== system Simulator/Mode 4: Slew1/Tcurrent ==
  Quaternion : Inport
  u : Inport  Port=2
  Clock : Clock
  Compare To Constant : simulink/Logic and Bit Operations/Compare To Constant  relop=>=  const=4.0  OutDataTypeStr=boolean
  Display{,1..3} (4 alike) : Display
  Enabled Subsystem : Subsystem  TreatAsAtomicUnit=on
  Subtract1 : Sum  Inputs=+-
  Out1 : Outport
  Output : Outport  Port=2
  Output1 : Outport  Port=3
  wires:
  Compare To Constant/1 -> Display/1, Enabled Subsystem/Enable
  Subtract1/1 -> Out1/1
  Enabled Subsystem/1(Out1) -> Subtract1/2, Output/1
  u/1 -> Display3/1, Compare To Constant/1
  Clock/1 -> Enabled Subsystem/2(In2), Subtract1/1
  Quaternion/1 -> Enabled Subsystem/1(In1), Display2/1
  Enabled Subsystem/2(Out2) -> Display1/1, Output1/1

== system Simulator/Mode 4: Slew1/w (q1,q2,q3,q0) to (q0,q1,q2,q3)  ==
  y : Inport
  Vector Concatenate : Concatenate
  e_q_vect1 : Selector  InputPortWidth=4  IndexOptions=Index vector (dialog)  Indices=[1 2 3]  OutputSizes=1
  e_q_vect2 : Selector  InputPortWidth=4  IndexOptions=Index vector (dialog)  Indices=[4]  OutputSizes=1
  Out1 : Outport
  wires:
  y/1 -> e_q_vect2/1, e_q_vect1/1
  e_q_vect2/1 -> Vector Concatenate/1
  e_q_vect1/1 -> Vector Concatenate/2
  Vector Concatenate/1 -> Out1/1

== system Simulator/Mode 5: Attitude Control/Free Rigid Body  ==
  torque command : Inport
  Cross : Subsystem
  Inertia : Gain  Gain=I  Multiplication=Matrix(K*u)  SaturateOnIntegerOverflow=on  OutDataTypeStr=Inherit: Same as input  ParamDataTypeStr=Inherit: Same as input
  Isc inverse : Gain  Gain=invI  Multiplication=Matrix(K*u)  SaturateOnIntegerOverflow=on  OutDataTypeStr=Inherit: Same as input  ParamDataTypeStr=Inherit: Same as input
  Quaternion Integration : Subsystem
  Sum : Sum  Inputs=|+-  InputSameDT=on  SaturateOnIntegerOverflow=on  OutDataTypeStr=Inherit: Same as first input
  "wdot -> w" : Integrator  InitialCondition=wbn_init
  q : Outport
  w : Outport  Port=2
  wires:
  Isc inverse/1 -> "wdot -> w"/1
  "wdot -> w"/1 -> w/1, Quaternion Integration/1(w_Body), Inertia/1, Cross/1(A)
  Sum/1 -> Isc inverse/1
  torque command/1 -> Sum/1
  Cross/1(AxB) -> Sum/2
  Inertia/1 -> Cross/2(B)
  Quaternion Integration/1(q_I_Body) -> q/1

== system Simulator/Mode 6: Momentum Dump/Cross ==
  A : Inport
  B : Inport  Port=2
  Mux4 : Mux  Inputs=3
  Product{,1..5} (6 alike) : Product  InputSameDT=on  SaturateOnIntegerOverflow=on  OutDataTypeStr=Inherit: Same as first input
  Sum : Sum  Inputs=+-  InputSameDT=on  SaturateOnIntegerOverflow=on  OutDataTypeStr=Inherit: Same as first input
  Sum1 : Sum  Inputs=+-  InputSameDT=on  SaturateOnIntegerOverflow=on  OutDataTypeStr=Inherit: Same as first input
  Sum2 : Sum  Inputs=+-  InputSameDT=on  SaturateOnIntegerOverflow=on  OutDataTypeStr=Inherit: Same as first input
  demux2 : Demux  Outputs=3
      settings: DisplayOption=none
  demux3 : Demux  Outputs=3
      settings: DisplayOption=none
  AxB : Outport  InitialOutput=0
  wires:
  A/1 -> demux2/1
  B/1 -> demux3/1
  demux2/3 -> Product1/1, Product2/1
  demux3/3 -> Product/2, Product3/2
  demux2/1 -> Product3/1, Product4/1
  demux3/2 -> Product1/2, Product4/2
  demux2/2 -> Product/1, Product5/1
  demux3/1 -> Product2/2, Product5/2
  Product/1 -> Sum/1
  Product1/1 -> Sum/2
  Product2/1 -> Sum1/1
  Product3/1 -> Sum1/2
  Product4/1 -> Sum2/1
  Product5/1 -> Sum2/2
  Sum/1 -> Mux4/1
  Sum1/1 -> Mux4/2
  Sum2/1 -> Mux4/3
  Mux4/1 -> AxB/1

== system Simulator/Mode 3: Constant Rate/Free Rigid Body /Cross ==
  A : Inport
  B : Inport  Port=2
  Mux4 : Mux  Inputs=3
  Product{,1..5} (6 alike) : Product  InputSameDT=on  SaturateOnIntegerOverflow=on  OutDataTypeStr=Inherit: Same as first input
  Sum : Sum  Inputs=+-  InputSameDT=on  SaturateOnIntegerOverflow=on  OutDataTypeStr=Inherit: Same as first input
  Sum1 : Sum  Inputs=+-  InputSameDT=on  SaturateOnIntegerOverflow=on  OutDataTypeStr=Inherit: Same as first input
  Sum2 : Sum  Inputs=+-  InputSameDT=on  SaturateOnIntegerOverflow=on  OutDataTypeStr=Inherit: Same as first input
  demux2 : Demux  Outputs=3
      settings: DisplayOption=none
  demux3 : Demux  Outputs=3
      settings: DisplayOption=none
  AxB : Outport  InitialOutput=0
  wires:
  A/1 -> demux2/1
  B/1 -> demux3/1
  demux2/3 -> Product1/1, Product2/1
  demux3/3 -> Product/2, Product3/2
  demux2/1 -> Product3/1, Product4/1
  demux3/2 -> Product1/2, Product4/2
  demux2/2 -> Product/1, Product5/1
  demux3/1 -> Product2/2, Product5/2
  Product/1 -> Sum/1
  Product1/1 -> Sum/2
  Product2/1 -> Sum1/1
  Product3/1 -> Sum1/2
  Product4/1 -> Sum2/1
  Product5/1 -> Sum2/2
  Sum/1 -> Mux4/1
  Sum1/1 -> Mux4/2
  Sum2/1 -> Mux4/3
  Mux4/1 -> AxB/1

== system Simulator/Mode 3: Constant Rate/Free Rigid Body /Quaternion Integration ==
  w_Body : Inport
  Integrator1 : Integrator  InitialCondition=q_init
  q_normalize : Subsystem
  qderiv : Subsystem
  q_I_Body : Outport
  wires:
  w_Body/1 -> qderiv/1(w)
  q_normalize/1(q_out) -> qderiv/2(q), q_I_Body/1
  Integrator1/1 -> q_normalize/1(q_in)
  qderiv/1(qd) -> Integrator1/1

== system Simulator/Mode 3: Constant Rate/Free Rigid Body /Subsystem ==
  q1 q2 q3 q4 : Inport
  Demux : Demux
      settings: DisplayOption=none
  Gain1 : Gain  Gain=2  SaturateOnIntegerOverflow=on  OutDataTypeStr=Inherit: Same as input  ParamDataTypeStr=Inherit: Same as input
  Gain2 : Gain  Gain=2  SaturateOnIntegerOverflow=on  OutDataTypeStr=Inherit: Same as input  ParamDataTypeStr=Inherit: Same as input
  Matrix Gain : Gain  Gain=eye(3,3)  SaturateOnIntegerOverflow=on  OutDataTypeStr=Inherit: Same as input  ParamDataTypeStr=Inherit: Same as input
  Mux : Mux  Inputs=3
  Product : Product  InputSameDT=on  SaturateOnIntegerOverflow=on  OutDataTypeStr=Inherit: Same as first input
  Product1 : Product  InputSameDT=on  SaturateOnIntegerOverflow=on  OutDataTypeStr=Inherit: Same as first input
  Subsystem : Subsystem
      mask Display: disp('3x3 cross matrix')
  Sum1 : Sum  Inputs=|+-  InputSameDT=on  SaturateOnIntegerOverflow=on  OutDataTypeStr=Inherit: Same as first input
  Sum8 : Sum  Inputs=|+-+  InputSameDT=on  SaturateOnIntegerOverflow=on  OutDataTypeStr=Inherit: Same as first input
  T1 : Math  Operator=transpose  SignedPower=on
  T2 : Math  Operator=transpose  SignedPower=on
  qTq : Product  Multiplication=Matrix(*)  InputSameDT=on  SaturateOnIntegerOverflow=on  OutDataTypeStr=Inherit: Same as first input
  qqT : Product  Multiplication=Matrix(*)  InputSameDT=on  SaturateOnIntegerOverflow=on  OutDataTypeStr=Inherit: Same as first input
  DCM : Outport  InitialOutput=0
  wires:
  T1/1 -> qqT/2
  Sum8/1 -> DCM/1
  Product/1 -> Gain1/1
  Demux/3 -> Mux/3
  Demux/2 -> Mux/2
  qqT/1 -> Gain2/1
  Gain1/1 -> Sum8/2
  q1 q2 q3 q4/1 -> Demux/1
  Demux/1 -> Mux/1
  Matrix Gain/1 -> Sum8/3
  Product1/1 -> Sum1/1
  qTq/1 -> Sum1/2
  T2/1 -> qTq/1
  Subsystem/1(Out1) -> Product/1
  Mux/1 -> qTq/2, T2/1, qqT/1, T1/1, Subsystem/1(In1)
  Demux/4 -> Product1/2, Product1/1, Product/2
  Sum1/1 -> Matrix Gain/1
  Gain2/1 -> Sum8/1

== system Simulator/Mode 4: Slew/Free Rigid Body 1/Cross ==
  A : Inport
  B : Inport  Port=2
  Mux4 : Mux  Inputs=3
  Product{,1..5} (6 alike) : Product  InputSameDT=on  SaturateOnIntegerOverflow=on  OutDataTypeStr=Inherit: Same as first input
  Sum : Sum  Inputs=+-  InputSameDT=on  SaturateOnIntegerOverflow=on  OutDataTypeStr=Inherit: Same as first input
  Sum1 : Sum  Inputs=+-  InputSameDT=on  SaturateOnIntegerOverflow=on  OutDataTypeStr=Inherit: Same as first input
  Sum2 : Sum  Inputs=+-  InputSameDT=on  SaturateOnIntegerOverflow=on  OutDataTypeStr=Inherit: Same as first input
  demux2 : Demux  Outputs=3
      settings: DisplayOption=none
  demux3 : Demux  Outputs=3
      settings: DisplayOption=none
  AxB : Outport  InitialOutput=0
  wires:
  A/1 -> demux2/1
  B/1 -> demux3/1
  demux2/3 -> Product1/1, Product2/1
  demux3/3 -> Product/2, Product3/2
  demux2/1 -> Product3/1, Product4/1
  demux3/2 -> Product1/2, Product4/2
  demux2/2 -> Product/1, Product5/1
  demux3/1 -> Product2/2, Product5/2
  Product/1 -> Sum/1
  Product1/1 -> Sum/2
  Product2/1 -> Sum1/1
  Product3/1 -> Sum1/2
  Product4/1 -> Sum2/1
  Product5/1 -> Sum2/2
  Sum/1 -> Mux4/1
  Sum1/1 -> Mux4/2
  Sum2/1 -> Mux4/3
  Mux4/1 -> AxB/1

== system Simulator/Mode 4: Slew/Free Rigid Body 1/Quaternion Integration ==
  w_Body : Inport
  Integrator1 : Integrator  InitialCondition=q_init
  q_normalize : Subsystem
  qderiv : Subsystem
  q_I_Body : Outport
  wires:
  w_Body/1 -> qderiv/1(w)
  q_normalize/1(q_out) -> qderiv/2(q), q_I_Body/1
  Integrator1/1 -> q_normalize/1(q_in)
  qderiv/1(qd) -> Integrator1/1

== system Simulator/Mode 4: Slew/Free Rigid Body 1/Subsystem ==
  q1 q2 q3 q4 : Inport
  Demux : Demux
      settings: DisplayOption=none
  Gain1 : Gain  Gain=2  SaturateOnIntegerOverflow=on  OutDataTypeStr=Inherit: Same as input  ParamDataTypeStr=Inherit: Same as input
  Gain2 : Gain  Gain=2  SaturateOnIntegerOverflow=on  OutDataTypeStr=Inherit: Same as input  ParamDataTypeStr=Inherit: Same as input
  Matrix Gain : Gain  Gain=eye(3,3)  SaturateOnIntegerOverflow=on  OutDataTypeStr=Inherit: Same as input  ParamDataTypeStr=Inherit: Same as input
  Mux : Mux  Inputs=3
  Product : Product  InputSameDT=on  SaturateOnIntegerOverflow=on  OutDataTypeStr=Inherit: Same as first input
  Product1 : Product  InputSameDT=on  SaturateOnIntegerOverflow=on  OutDataTypeStr=Inherit: Same as first input
  Subsystem : Subsystem
      mask Display: disp('3x3 cross matrix')
  Sum1 : Sum  Inputs=|+-  InputSameDT=on  SaturateOnIntegerOverflow=on  OutDataTypeStr=Inherit: Same as first input
  Sum8 : Sum  Inputs=|+-+  InputSameDT=on  SaturateOnIntegerOverflow=on  OutDataTypeStr=Inherit: Same as first input
  T1 : Math  Operator=transpose  SignedPower=on
  T2 : Math  Operator=transpose  SignedPower=on
  qTq : Product  Multiplication=Matrix(*)  InputSameDT=on  SaturateOnIntegerOverflow=on  OutDataTypeStr=Inherit: Same as first input
  qqT : Product  Multiplication=Matrix(*)  InputSameDT=on  SaturateOnIntegerOverflow=on  OutDataTypeStr=Inherit: Same as first input
  DCM : Outport  InitialOutput=0
  wires:
  T1/1 -> qqT/2
  Sum8/1 -> DCM/1
  Product/1 -> Gain1/1
  Demux/3 -> Mux/3
  Demux/2 -> Mux/2
  qqT/1 -> Gain2/1
  Gain1/1 -> Sum8/2
  q1 q2 q3 q4/1 -> Demux/1
  Demux/1 -> Mux/1
  Matrix Gain/1 -> Sum8/3
  Product1/1 -> Sum1/1
  qTq/1 -> Sum1/2
  T2/1 -> qTq/1
  Subsystem/1(Out1) -> Product/1
  Mux/1 -> qTq/2, T2/1, qqT/1, T1/1, Subsystem/1(In1)
  Demux/4 -> Product1/2, Product1/1, Product/2
  Sum1/1 -> Matrix Gain/1
  Gain2/1 -> Sum8/1

== system Simulator/Mode 4: Slew1/ACS/Free Rigid Body  ==
  torque command : Inport
  Cross : Subsystem
  Inertia : Gain  Gain=I  Multiplication=Matrix(K*u)  SaturateOnIntegerOverflow=on  OutDataTypeStr=Inherit: Same as input  ParamDataTypeStr=Inherit: Same as input
  Isc inverse : Gain  Gain=invI  Multiplication=Matrix(K*u)  SaturateOnIntegerOverflow=on  OutDataTypeStr=Inherit: Same as input  ParamDataTypeStr=Inherit: Same as input
  Quaternion Integration : Subsystem
  Sum : Sum  Inputs=|+-  InputSameDT=on  SaturateOnIntegerOverflow=on  OutDataTypeStr=Inherit: Same as first input
  "wdot -> w" : Integrator  InitialCondition=wbn_init
  q : Outport
  w : Outport  Port=2
  wires:
  Isc inverse/1 -> "wdot -> w"/1
  "wdot -> w"/1 -> w/1, Quaternion Integration/1(w_Body), Inertia/1, Cross/1(A)
  Sum/1 -> Isc inverse/1
  torque command/1 -> Sum/1
  Cross/1(AxB) -> Sum/2
  Inertia/1 -> Cross/2(B)
  Quaternion Integration/1(q_I_Body) -> q/1

== system Simulator/Mode 4: Slew1/DCM to Axis-Angle/a1 ==
  In1 : Inport
  Input : Inport  Port=2
  phi : Inport  Port=3
  Divide : Product  Inputs=*/
  Minus : Sum  Inputs=+-
  Multiply : Gain  Gain=2
  Sin : Trigonometry
  a1 : Outport
  wires:
  In1/1 -> Minus/1
  Input/1 -> Minus/2
  phi/1 -> Sin/1
  Sin/1 -> Multiply/1
  Minus/1 -> Divide/1
  Divide/1 -> a1/1
  Multiply/1 -> Divide/2

== system Simulator/Mode 4: Slew1/DCM to Axis-Angle/a2 ==
  In1 : Inport
  Input : Inport  Port=2
  phi : Inport  Port=3
  Divide : Product  Inputs=*/
  Minus : Sum  Inputs=+-
  Multiply : Gain  Gain=2
  Sin : Trigonometry
  a2 : Outport
  wires:
  In1/1 -> Minus/1
  Input/1 -> Minus/2
  phi/1 -> Sin/1
  Sin/1 -> Multiply/1
  Minus/1 -> Divide/1
  Divide/1 -> a2/1
  Multiply/1 -> Divide/2

== system Simulator/Mode 4: Slew1/DCM to Axis-Angle/a3 ==
  In1 : Inport
  Input : Inport  Port=2
  phi : Inport  Port=3
  Divide : Product  Inputs=*/
  Minus : Sum  Inputs=+-
  Multiply : Gain  Gain=2
  Sin : Trigonometry
  a3 : Outport
  wires:
  In1/1 -> Minus/1
  Input/1 -> Minus/2
  phi/1 -> Sin/1
  Sin/1 -> Multiply/1
  Minus/1 -> Divide/1
  Divide/1 -> a3/1
  Multiply/1 -> Divide/2

== system Simulator/Mode 4: Slew1/DCM to Axis-Angle/phi ==
  In1 : Inport
  Input : Inport  Port=2
  Input1 : Inport  Port=3
  Acos : Trigonometry  Operator=acos
  Add : Sum  Inputs=++++
  Constant : Constant  Value=-1
  Multiply : Gain  Gain=0.5
  phi : Outport
  wires:
  Input1/1 -> Add/3
  Input/1 -> Add/2
  In1/1 -> Add/1
  Constant/1 -> Add/4
  Add/1 -> Multiply/1
  Multiply/1 -> Acos/1
  Acos/1 -> phi/1

== system Simulator/Mode 4: Slew1/DCM to Axis-Angle1/a1 ==
  In1 : Inport
  Input : Inport  Port=2
  phi : Inport  Port=3
  Divide : Product  Inputs=*/
  Minus : Sum  Inputs=+-
  Multiply : Gain  Gain=2
  Sin : Trigonometry
  a1 : Outport
  wires:
  Multiply/1 -> Divide/2
  Divide/1 -> a1/1
  Minus/1 -> Divide/1
  Sin/1 -> Multiply/1
  phi/1 -> Sin/1
  Input/1 -> Minus/2
  In1/1 -> Minus/1

== system Simulator/Mode 4: Slew1/DCM to Axis-Angle1/a2 ==
  In1 : Inport
  Input : Inport  Port=2
  phi : Inport  Port=3
  Divide : Product  Inputs=*/
  Minus : Sum  Inputs=+-
  Multiply : Gain  Gain=2
  Sin : Trigonometry
  a2 : Outport
  wires:
  Multiply/1 -> Divide/2
  Divide/1 -> a2/1
  Minus/1 -> Divide/1
  Sin/1 -> Multiply/1
  phi/1 -> Sin/1
  Input/1 -> Minus/2
  In1/1 -> Minus/1

== system Simulator/Mode 4: Slew1/DCM to Axis-Angle1/a3 ==
  In1 : Inport
  Input : Inport  Port=2
  phi : Inport  Port=3
  Divide : Product  Inputs=*/
  Minus : Sum  Inputs=+-
  Multiply : Gain  Gain=2
  Sin : Trigonometry
  a3 : Outport
  wires:
  Multiply/1 -> Divide/2
  Divide/1 -> a3/1
  Minus/1 -> Divide/1
  Sin/1 -> Multiply/1
  phi/1 -> Sin/1
  Input/1 -> Minus/2
  In1/1 -> Minus/1

== system Simulator/Mode 4: Slew1/DCM to Axis-Angle1/phi ==
  In1 : Inport
  Input : Inport  Port=2
  Input1 : Inport  Port=3
  Acos : Trigonometry  Operator=acos
  Add : Sum  Inputs=++++
  Constant : Constant  Value=-1
  Multiply : Gain  Gain=0.5
  phi : Outport
  wires:
  Acos/1 -> phi/1
  Multiply/1 -> Acos/1
  Add/1 -> Multiply/1
  Constant/1 -> Add/4
  In1/1 -> Add/1
  Input/1 -> Add/2
  Input1/1 -> Add/3

== system Simulator/Mode 4: Slew1/Subsystem/Quaternion Integration ==
  w_Body : Inport
  Integrator1 : Integrator  InitialCondition=q_init
  q_normalize : Subsystem
  qderiv : Subsystem
  q_I_Body : Outport
  wires:
  qderiv/1(qd) -> Integrator1/1
  Integrator1/1 -> q_normalize/1(q_in)
  q_normalize/1(q_out) -> q_I_Body/1, qderiv/2(q)
  w_Body/1 -> qderiv/1(w)

== system Simulator/Mode 4: Slew1/Subsystem/S ==
  Input : Inport
  Divide : Product  Inputs=*/
  Pi1 : Constant  Value=pi  OutDataTypeStr=Inherit: Inherit via back propagation
  Subtract1 : Sum  Commented=on  Inputs=+-
  "Total time " : Constant  Value=300
  Out1 : Outport
  wires:
  Divide/1 -> Out1/1
  Pi1/1 -> Divide/1
  Input/1 -> Subtract1/2
  "Total time "/1 -> Divide/2

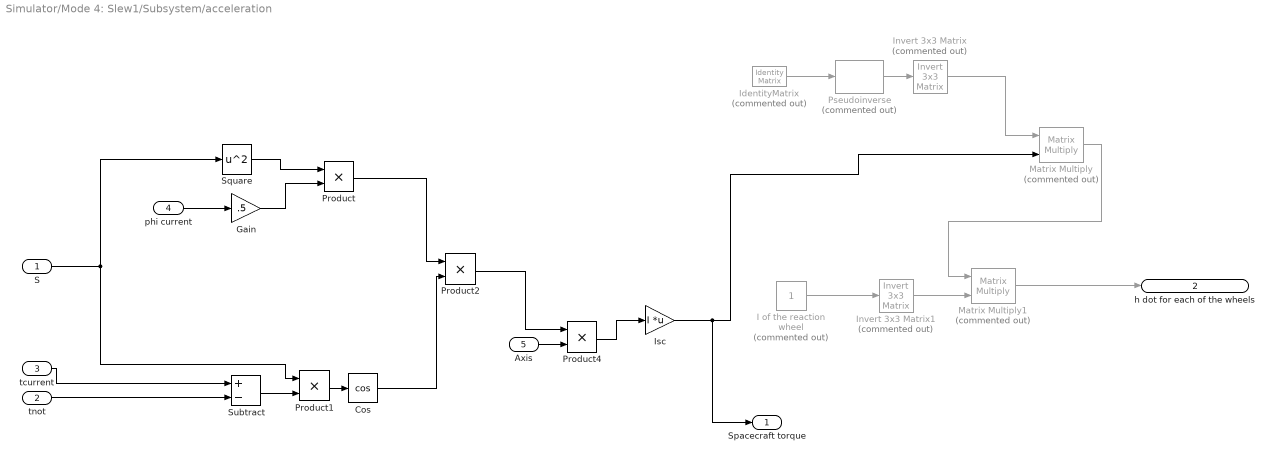
== system Simulator/Mode 4: Slew1/Subsystem/acceleration ==
  S : Inport
  tnot : Inport  Port=2
  tcurrent : Inport  Port=3
  phi current : Inport  Port=4
  Axis : Inport  Port=5
  Cos : Trigonometry  Operator=cos
  Gain : Gain  Gain=.5
  I of the reaction wheel : Constant  Commented=on
  IdentityMatrix : IdentityMatrix  Commented=on  OutputDimensions=3
  Invert 3x3 Matrix : aerolibutil/Invert  3x3 Matrix  Commented=on
  Invert 3x3 Matrix1 : aerolibutil/Invert  3x3 Matrix  Commented=on
  Isc : Gain  Gain=I  Multiplication=Matrix(K*u)
  Matrix Multiply : Product  Commented=on  Multiplication=Matrix(*)
  Matrix Multiply1 : Product  Commented=on  Multiplication=Matrix(*)
  Product{,1..2,4} (4 alike) : Product
  Pseudoinverse : dspinverses/Pseudoinverse  Commented=on  wanterr=off  SimulateUsing=Interpreted execution
  Square : Math  Operator=square
  Subtract : Sum  Inputs=+-
  Spacecraft torque : Outport
  h dot for each of the wheels : Outport  Port=2
  wires:
  S/1 -> Square/1, Product1/1
  Square/1 -> Product/1
  phi current/1 -> Gain/1
  Gain/1 -> Product/2
  tcurrent/1 -> Subtract/1
  tnot/1 -> Subtract/2
  Subtract/1 -> Product1/2
  Product1/1 -> Cos/1
  Product/1 -> Product2/1
  IdentityMatrix/1 -> Pseudoinverse/1
  Pseudoinverse/1 -> Invert 3x3 Matrix/1
  Invert 3x3 Matrix/1 -> Matrix Multiply/1
  Isc/1 -> Matrix Multiply/2, Spacecraft torque/1
  I of the reaction wheel/1 -> Invert 3x3 Matrix1/1
  Matrix Multiply/1 -> Matrix Multiply1/1
  Invert 3x3 Matrix1/1 -> Matrix Multiply1/2
  Cos/1 -> Product2/2
  Product2/1 -> Product4/1
  Axis/1 -> Product4/2
  Product4/1 -> Isc/1
  Matrix Multiply1/1 -> h dot for each of the wheels/1

== system Simulator/Mode 4: Slew1/Subsystem2/Enabled Subsystem ==
  In1 : Inport
  Enable : EnablePort
  Out1 : Outport
  wires:
  In1/1 -> Out1/1

== system Simulator/Mode 4: Slew1/Subsystem2/Subsystem ==
  Input : Inport
  Quaternions to Direction Cosine Matrix2 : sharedtransform/Quaternions to  Direction Cosine Matrix  aMode=aMode
      settings: LibrarySourceBlock=|
      | aerolibtransform2/Quaternions to
      | Direction Cosine Matrix
  Subsystem3 : Subsystem
  "w (q1,q2,q3,q0) to (q0,q1,q2,q3) " : Subsystem
      settings: PortSchema="{\"entries\":[{\"content\":{\"sides\":[{\"content\":{\"connectorIds\":[\"Out1\"]},\"type\":\"ConnectorPlacement.EquallySpacedRectSide\",\"uuid\":\"97b477ad-5663-4010-b344-d27b8ec095be\"},{\"content\":{\"connectorIds\":[\"In1\"],\"side\":\"RIGHT\"},\"type\":\"ConnectorPlacement.EquallySpacedRectSide\",\"uuid\":\"41fe4029-0263-4427-bdfc-3c26258b8a65\"},{\"content\":{\"side\":\"TOP\"},\"type\":\"ConnectorPlacement.EquallySpacedRectSide\",\"uuid\":\"9fb3a03d-539a-4245-bd7d-8174d3d0797f\"}]},\"type\":\"ConnectorPlacement.EquallySpacedConnector\",\"uuid\":\"44222554-f3ae-4bc6-b92c-7571a5ce84f7\"}],\"packageUris\":[\"http://schema.mathworks.com/mf0/Connector/R2020b\"],\"version\":\"1.0\"}"
  Angle (phi) : Outport
  wires:
  Quaternions to Direction Cosine Matrix2/1 -> Subsystem3/1(In1)
  Input/1 -> "w (q1,q2,q3,q0) to (q0,q1,q2,q3) "/1(y)
  Subsystem3/2(Angle (phi)) -> Angle (phi)/1
  "w (q1,q2,q3,q0) to (q0,q1,q2,q3) "/1(Out1) -> Quaternions to Direction Cosine Matrix2/1

== system Simulator/Mode 4: Slew1/Tcurrent/Enabled Subsystem ==
  In1 : Inport
  In2 : Inport  Port=2
  Enable : EnablePort
  Out1 : Outport
  Out2 : Outport  Port=2
  wires:
  In1/1 -> Out1/1

== system Simulator/Mode 5: Attitude Control/Free Rigid Body /Cross ==
  A : Inport
  B : Inport  Port=2
  Mux4 : Mux  Inputs=3
  Product{,1..5} (6 alike) : Product  InputSameDT=on  SaturateOnIntegerOverflow=on  OutDataTypeStr=Inherit: Same as first input
  Sum : Sum  Inputs=+-  InputSameDT=on  SaturateOnIntegerOverflow=on  OutDataTypeStr=Inherit: Same as first input
  Sum1 : Sum  Inputs=+-  InputSameDT=on  SaturateOnIntegerOverflow=on  OutDataTypeStr=Inherit: Same as first input
  Sum2 : Sum  Inputs=+-  InputSameDT=on  SaturateOnIntegerOverflow=on  OutDataTypeStr=Inherit: Same as first input
  demux2 : Demux  Outputs=3
      settings: DisplayOption=none
  demux3 : Demux  Outputs=3
      settings: DisplayOption=none
  AxB : Outport  InitialOutput=0
  wires:
  A/1 -> demux2/1
  B/1 -> demux3/1
  demux2/3 -> Product1/1, Product2/1
  demux3/3 -> Product/2, Product3/2
  demux2/1 -> Product3/1, Product4/1
  demux3/2 -> Product1/2, Product4/2
  demux2/2 -> Product/1, Product5/1
  demux3/1 -> Product2/2, Product5/2
  Product/1 -> Sum/1
  Product1/1 -> Sum/2
  Product2/1 -> Sum1/1
  Product3/1 -> Sum1/2
  Product4/1 -> Sum2/1
  Product5/1 -> Sum2/2
  Sum/1 -> Mux4/1
  Sum1/1 -> Mux4/2
  Sum2/1 -> Mux4/3
  Mux4/1 -> AxB/1

== system Simulator/Mode 5: Attitude Control/Free Rigid Body /Quaternion Integration ==
  w_Body : Inport
  Integrator1 : Integrator  InitialCondition=q_init
  q_normalize : Subsystem
  qderiv : Subsystem
  q_I_Body : Outport
  wires:
  w_Body/1 -> qderiv/1(w)
  q_normalize/1(q_out) -> qderiv/2(q), q_I_Body/1
  Integrator1/1 -> q_normalize/1(q_in)
  qderiv/1(qd) -> Integrator1/1

== system Simulator/Mode 3: Constant Rate/Free Rigid Body /Quaternion Integration/q_normalize ==
  q_in : Inport  PortDimensions=4
  Dot Product : DotProduct  OutDataTypeStr=Inherit: Inherit via internal rule
  Product : Product  Inputs=*/  InputSameDT=on  SaturateOnIntegerOverflow=on  OutDataTypeStr=Inherit: Same as first input
  SignedSqrt : Sqrt  IntermediateResultsDataTypeStr=double
  q_out : Outport
  wires:
  Product/1 -> q_out/1
  SignedSqrt/1 -> Product/2
  q_in/1 -> Dot Product/2, Dot Product/1, Product/1
  Dot Product/1 -> SignedSqrt/1
